simulink model "sim_project2"  (R2022a)
settings: Solver=VariableStepAuto  StartTime=0.0  StopTime=10.0  RelTol=1e-3
values from neighbouring files (symbols this model uses):
  A = A-B*Kctrl    [project.m]
  Ad = [0 0 0 0 0 0; 1 0 0 0 0 0; 2 1 0 0 0 0; 3 1 6 0 0 0; 1 2 1 3 0 0; 1 1 1 4 1 0]    [project.m]
  B = [0 -9.9453]'    [project.m]
  C = [708.27 0; 0 0]    [project.m]
  c = 10/(2*min(real(lam_g)))    [project.m]
  F = -F'    [project.m]
  G = diag([1 1 1 1 1 1])    [project.m]
  K = R^-1*B'*Pc    [project.m]
  Lun = Lun'    [project.m]
  n = length(B)    [project.m]
  noise = randn    [project.m]
  X0 = [10 2]'    [project.m]
settings Model: Creator=matildezampolini  LastModifiedBy=matildezampolini

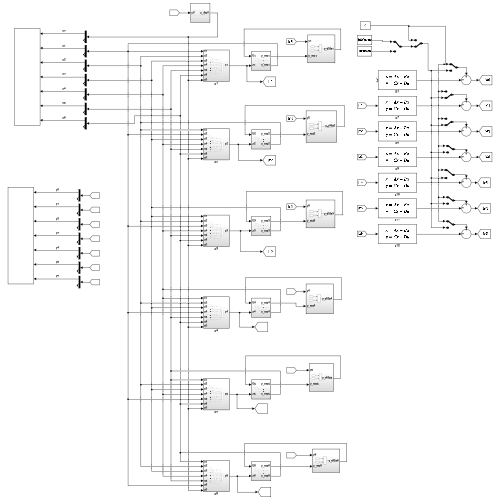
[thumbnail: Simulink's stored preview of the top-level diagram]
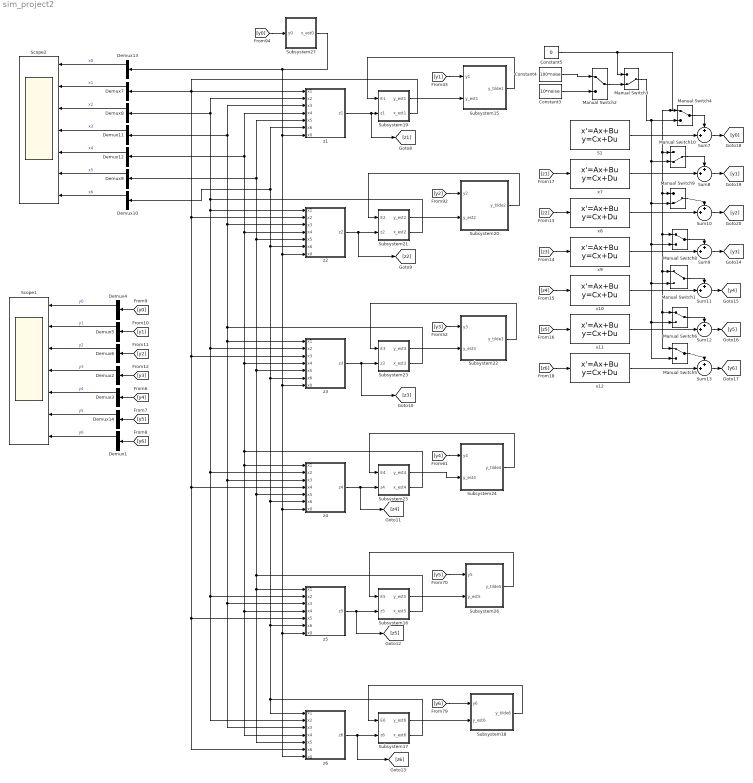
== system sim_project2 ==
  Constant3 : Constant  Value=10*noise
  Constant4 : Constant  Value=100*noise
  Constant5 : Constant  Value=0
  Demux{1..14} (14 alike) : Demux  Outputs=2
  Manual Switch{1..2,4..6,8} (6 alike) : ManualSwitch
  Manual Switch10 : ManualSwitch  CurrentSetting=0
  Manual Switch3 : ManualSwitch  CurrentSetting=0
  Manual Switch9 : ManualSwitch  CurrentSetting=0
  S1 : StateSpace  A=A  B=zeros(n,1)  C=C  D=zeros(n,1)  InitialCondition=X0
  Scope1 : Scope  NumInputPorts=7
  Scope2 : Scope  NumInputPorts=7
  Subsystem15 : Subsystem
  Subsystem16 : Subsystem
  Subsystem17 : Subsystem
  Subsystem18 : Subsystem
  Subsystem19 : Subsystem
  Subsystem20 : Subsystem
  Subsystem21 : Subsystem
  Subsystem22 : Subsystem
  Subsystem23 : Subsystem
  Subsystem24 : Subsystem
  Subsystem25 : Subsystem
  Subsystem26 : Subsystem
  Subsystem27 : Subsystem
  Sum{7..13} (7 alike) : Sum  Inputs=++|
  x{7..12} (6 alike) : StateSpace  A=A  B=c*B*K  C=C  D=zeros(n)  InitialCondition=0
  z1 : Subsystem
  z2 : Subsystem
  z3 : Subsystem
  z4 : Subsystem
  z5 : Subsystem
  z6 : Subsystem
  wires:
  [y4] -> Subsystem24/1(y4)
  Demux14/1 -> Scope1/6  "y5"
  Subsystem19/2(x_est1) -> Demux7/1, z2/2(x2), z5/5(x5), z6/6(x6), z4/4(x4), z3/3(x3), z1/1(x1)
  [y2] -> Demux6/1
  [y5] -> Subsystem26/1(y5)
  z5/1(z5) -> [z5], Subsystem16/2(z5)
  z1/1(z1) -> [z1], Subsystem19/2(z1)
  Subsystem25/1(y_est4) -> Subsystem24/2(y_est4)
  Demux4/1 -> Scope1/1  "y0"
  z6/1(z6) -> [z6], Subsystem17/2(z6)
  Demux5/1 -> Scope1/2  "y1"
  Demux3/1 -> Scope1/5  "y4"
  Subsystem25/2(x_est4) -> z3/4(x4), z2/4(x4), Demux12/1, z1/4(x4), z4/1(x1), z6/4(x4), z5/4(x4)
  Subsystem23/1(y_est3) -> Subsystem22/2(y_est3)
  Demux1/1 -> Scope1/7  "y6"
  Demux12/1 -> Scope2/5  "x4"
  Subsystem21/2(x_est2) -> z2/1(x1), z4/2(x2), z5/2(x2), z6/2(x2), z3/2(x2), z1/2(x2), Demux8/1
  Subsystem23/2(x_est3) -> z3/1(x1), z4/3(x3), z5/3(x3), z6/3(x3), z2/3(x3), Demux11/1, z1/3(x3)
  Demux9/1 -> Scope2/6  "x5"
  Demux6/1 -> Scope1/3  "y2"
  z4/1(z4) -> [z4], Subsystem25/2(z4)
  [y4] -> Demux3/1
  [y3] -> Demux2/1
  Demux2/1 -> Scope1/4  "y3"
  Subsystem16/1(y_est5) -> Subsystem26/2(y_est5)
  [y0] -> Demux4/1
  Subsystem17/2(x_est6) -> z5/6(x6), z3/6(x6), z2/6(x6), Demux10/1, z1/6(x6), z4/6(x6), z6/1(x1)
  [y6] -> Demux1/1
  [y1] -> Demux5/1
  [y5] -> Demux14/1
  Subsystem27/1(x_est0) -> z1/7(x0), z4/7(x0), z5/7(x0), z6/7(x0), z3/7(x0), z2/7(x0), Demux13/1
  [y1] -> Subsystem15/1(y1)
  Demux10/1 -> Scope2/7  "x6"
  Demux7/1 -> Scope2/2  "x1"
  Demux13/1 -> Scope2/1  "x0"
  [y3] -> Subsystem22/1(y3)
  Demux11/1 -> Scope2/4  "x3"
  [y2] -> Subsystem20/1(y2)
  Subsystem17/1(y_est6) -> Subsystem18/2(y_est6)
  Subsystem16/2(x_est5) -> z4/5(x5), z3/5(x5), z2/5(x5), z1/5(x5), Demux9/1, z5/1(x1), z6/5(x5)
  [y6] -> Subsystem18/1(y6)
  z3/1(z3) -> [z3], Subsystem23/2(z3)
  [y0] -> Subsystem27/1(y0)
  Subsystem21/1(y_est2) -> Subsystem20/2(y_est2)
  z2/1(z2) -> [z2], Subsystem21/2(z2)
  Demux8/1 -> Scope2/3  "x2"
  Subsystem19/1(y_est1) -> Subsystem15/2(y_est1)
  Subsystem15/1(y_tilde1) -> Subsystem19/1(E1)
  Subsystem20/1(y_tilde2) -> Subsystem21/1(E2)
  Subsystem22/1(y_tilde3) -> Subsystem23/1(E3)
  Subsystem24/1(y_tilde4) -> Subsystem25/1(E4)
  Subsystem26/1(y_tilde5) -> Subsystem16/1(E5)
  Subsystem18/1(y_tilde6) -> Subsystem17/1(E6)
  Manual Switch8/1 -> Sum9/1
  Sum8/1 -> [y1]
  [z4] -> x10/1
  Sum9/1 -> [y3]
  Sum10/1 -> [y2]
  [z5] -> x11/1
  Manual Switch4/1 -> Sum7/1
  [z2] -> x8/1
  Manual Switch10/1 -> Sum8/1
  Sum12/1 -> [y5]
  Manual Switch2/1 -> Manual Switch3/2
  [z3] -> x9/1
  Constant4/1 -> Manual Switch2/1
  Manual Switch3/1 -> Manual Switch4/2, Manual Switch8/2, Manual Switch1/2, Manual Switch6/2, Manual Switch5/2, Manual Switch9/2, Manual Switch10/2
  Manual Switch9/1 -> Sum10/1
  Manual Switch6/1 -> Sum12/1
  S1/1 -> Sum7/2
  x10/1 -> Sum11/2
  x12/1 -> Sum13/2
  [z6] -> x12/1
  x11/1 -> Sum12/2
  Manual Switch5/1 -> Sum13/1
  Manual Switch1/1 -> Sum11/1
  x7/1 -> Sum8/2
  Constant3/1 -> Manual Switch2/2
  x9/1 -> Sum9/2
  [z1] -> x7/1
  Constant5/1 -> Manual Switch1/1, Manual Switch5/1, Manual Switch6/1, Manual Switch8/1, Manual Switch9/1, Manual Switch10/1, Manual Switch4/1, Manual Switch3/1
  x8/1 -> Sum10/2
  Sum11/1 -> [y4]
  Sum7/1 -> [y0]
  Sum13/1 -> [y6]

== system sim_project2/Subsystem15 ==
  y1 : Inport
  y_est1 : Inport  Port=2
  Add2 : Sum  Inputs=+-
  y_tilde1 : Outport
  wires:
  Add2/1 -> y_tilde1/1
  y_est1/1 -> Add2/2
  y1/1 -> Add2/1

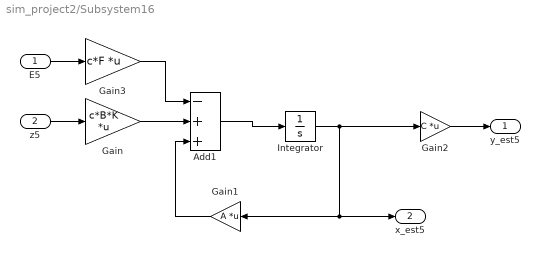
== system sim_project2/Subsystem16 ==
  E5 : Inport
  z5 : Inport  Port=2
  Add1 : Sum  Inputs=-++
  Gain : Gain  Gain=c*B*K  Multiplication=Matrix(K*u)
  Gain1 : Gain  Gain=A  Multiplication=Matrix(K*u)
  Gain2 : Gain  Gain=C  Multiplication=Matrix(K*u)
  Gain3 : Gain  Gain=c*F  Multiplication=Matrix(K*u)
  Integrator : Integrator
  y_est5 : Outport
  x_est5 : Outport  Port=2
  wires:
  Gain1/1 -> Add1/3
  E5/1 -> Gain3/1
  Add1/1 -> Integrator/1
  Gain3/1 -> Add1/1
  Gain2/1 -> y_est5/1
  Integrator/1 -> Gain2/1, x_est5/1, Gain1/1
  Gain/1 -> Add1/2
  z5/1 -> Gain/1

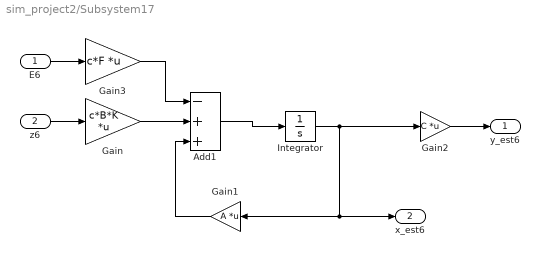
== system sim_project2/Subsystem17 ==
  E6 : Inport
  z6 : Inport  Port=2
  Add1 : Sum  Inputs=-++
  Gain : Gain  Gain=c*B*K  Multiplication=Matrix(K*u)
  Gain1 : Gain  Gain=A  Multiplication=Matrix(K*u)
  Gain2 : Gain  Gain=C  Multiplication=Matrix(K*u)
  Gain3 : Gain  Gain=c*F  Multiplication=Matrix(K*u)
  Integrator : Integrator
  y_est6 : Outport
  x_est6 : Outport  Port=2
  wires:
  Gain1/1 -> Add1/3
  E6/1 -> Gain3/1
  Add1/1 -> Integrator/1
  Gain3/1 -> Add1/1
  Gain2/1 -> y_est6/1
  Integrator/1 -> Gain2/1, x_est6/1, Gain1/1
  Gain/1 -> Add1/2
  z6/1 -> Gain/1

== system sim_project2/Subsystem18 ==
  y6 : Inport
  y_est6 : Inport  Port=2
  Add7 : Sum  Inputs=+-
  y_tilde6 : Outport
  wires:
  y_est6/1 -> Add7/2
  Add7/1 -> y_tilde6/1
  y6/1 -> Add7/1

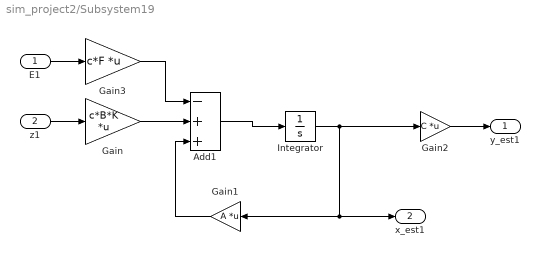
== system sim_project2/Subsystem19 ==
  E1 : Inport
  z1 : Inport  Port=2
  Add1 : Sum  Inputs=-++
  Gain : Gain  Gain=c*B*K  Multiplication=Matrix(K*u)
  Gain1 : Gain  Gain=A  Multiplication=Matrix(K*u)
  Gain2 : Gain  Gain=C  Multiplication=Matrix(K*u)
  Gain3 : Gain  Gain=c*F  Multiplication=Matrix(K*u)
  Integrator : Integrator
  y_est1 : Outport
  x_est1 : Outport  Port=2
  wires:
  E1/1 -> Gain3/1
  Add1/1 -> Integrator/1
  Gain3/1 -> Add1/1
  Gain2/1 -> y_est1/1
  Integrator/1 -> Gain2/1, x_est1/1, Gain1/1
  Gain/1 -> Add1/2
  z1/1 -> Gain/1
  Gain1/1 -> Add1/3

== system sim_project2/Subsystem20 ==
  y2 : Inport
  y_est2 : Inport  Port=2
  Add3 : Sum  Inputs=+-
  y_tilde2 : Outport
  wires:
  y_est2/1 -> Add3/2
  Add3/1 -> y_tilde2/1
  y2/1 -> Add3/1

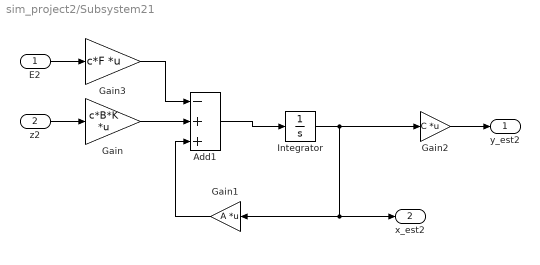
== system sim_project2/Subsystem21 ==
  E2 : Inport
  z2 : Inport  Port=2
  Add1 : Sum  Inputs=-++
  Gain : Gain  Gain=c*B*K  Multiplication=Matrix(K*u)
  Gain1 : Gain  Gain=A  Multiplication=Matrix(K*u)
  Gain2 : Gain  Gain=C  Multiplication=Matrix(K*u)
  Gain3 : Gain  Gain=c*F  Multiplication=Matrix(K*u)
  Integrator : Integrator
  y_est2 : Outport
  x_est2 : Outport  Port=2
  wires:
  E2/1 -> Gain3/1
  Add1/1 -> Integrator/1
  Gain3/1 -> Add1/1
  Gain2/1 -> y_est2/1
  Integrator/1 -> Gain2/1, x_est2/1, Gain1/1
  Gain/1 -> Add1/2
  z2/1 -> Gain/1
  Gain1/1 -> Add1/3

== system sim_project2/Subsystem22 ==
  y3 : Inport
  y_est3 : Inport  Port=2
  Add4 : Sum  Inputs=+-
  y_tilde3 : Outport
  wires:
  y_est3/1 -> Add4/2
  y3/1 -> Add4/1
  Add4/1 -> y_tilde3/1

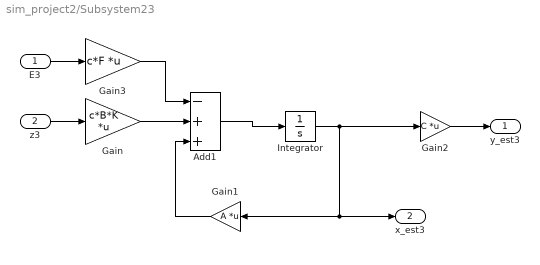
== system sim_project2/Subsystem23 ==
  E3 : Inport
  z3 : Inport  Port=2
  Add1 : Sum  Inputs=-++
  Gain : Gain  Gain=c*B*K  Multiplication=Matrix(K*u)
  Gain1 : Gain  Gain=A  Multiplication=Matrix(K*u)
  Gain2 : Gain  Gain=C  Multiplication=Matrix(K*u)
  Gain3 : Gain  Gain=c*F  Multiplication=Matrix(K*u)
  Integrator : Integrator
  y_est3 : Outport
  x_est3 : Outport  Port=2
  wires:
  E3/1 -> Gain3/1
  Add1/1 -> Integrator/1
  Gain3/1 -> Add1/1
  Gain2/1 -> y_est3/1
  Integrator/1 -> Gain2/1, x_est3/1, Gain1/1
  Gain/1 -> Add1/2
  z3/1 -> Gain/1
  Gain1/1 -> Add1/3

== system sim_project2/Subsystem24 ==
  y4 : Inport
  y_est4 : Inport  Port=2
  Add5 : Sum  Inputs=+-
  y_tilde4 : Outport
  wires:
  y_est4/1 -> Add5/2
  Add5/1 -> y_tilde4/1
  y4/1 -> Add5/1

== system sim_project2/Subsystem25 ==
  E4 : Inport
  z4 : Inport  Port=2
  Add1 : Sum  Inputs=-++
  Gain : Gain  Gain=c*B*K  Multiplication=Matrix(K*u)
  Gain1 : Gain  Gain=A  Multiplication=Matrix(K*u)
  Gain2 : Gain  Gain=C  Multiplication=Matrix(K*u)
  Gain3 : Gain  Gain=c*F  Multiplication=Matrix(K*u)
  Integrator : Integrator
  y_est4 : Outport
  x_est4 : Outport  Port=2
  wires:
  Gain1/1 -> Add1/3
  E4/1 -> Gain3/1
  Add1/1 -> Integrator/1
  Gain3/1 -> Add1/1
  Gain2/1 -> y_est4/1
  Integrator/1 -> Gain2/1, x_est4/1, Gain1/1
  Gain/1 -> Add1/2
  z4/1 -> Gain/1

== system sim_project2/Subsystem26 ==
  y5 : Inport
  y_est5 : Inport  Port=2
  Add6 : Sum  Inputs=+-
  y_tilde5 : Outport
  wires:
  Add6/1 -> y_tilde5/1
  y_est5/1 -> Add6/2
  y5/1 -> Add6/1

== system sim_project2/Subsystem27 ==
  y0 : Inport
  Add1 : Sum  Inputs=-+
  Add2 : Sum  Inputs=-+
  Gain1 : Gain  Gain=A  Multiplication=Matrix(K*u)
  Gain2 : Gain  Gain=C  Multiplication=Matrix(K*u)
  Gain4 : Gain  Gain=Lun  Multiplication=Matrix(K*u)
  Integrator : Integrator  InitialCondition=X0
  x_est0 : Outport
  wires:
  Add1/1 -> Integrator/1
  Gain2/1 -> Add2/2
  Integrator/1 -> Gain2/1, x_est0/1, Gain1/1
  y0/1 -> Add2/1
  Gain4/1 -> Add1/1
  Add2/1 -> Gain4/1
  Gain1/1 -> Add1/2

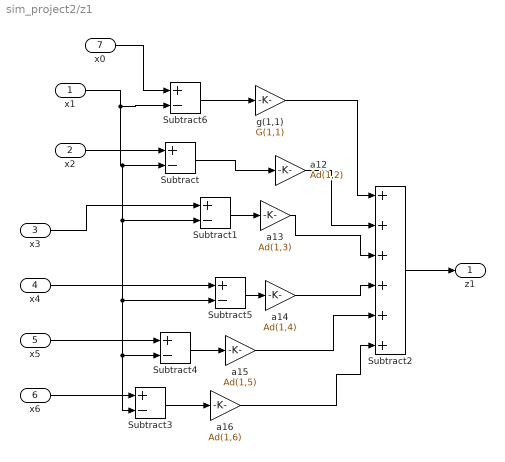
== system sim_project2/z1 ==
  x1 : Inport
  x2 : Inport  Port=2
  x3 : Inport  Port=3
  x4 : Inport  Port=4
  x5 : Inport  Port=5
  x6 : Inport  Port=6
  x0 : Inport  Port=7
  Subtract{,1,3..6} (6 alike) : Sum  Inputs=+-
  Subtract2 : Sum  Inputs=++++++
  a12 : Gain  Gain=Ad(1,2)
  a13 : Gain  Gain=Ad(1,3)
  a14 : Gain  Gain=Ad(1,4)
  a15 : Gain  Gain=Ad(1,5)
  a16 : Gain  Gain=Ad(1,6)
  g(1,1) : Gain  Gain=G(1,1)
  z1 : Outport
  wires:
  x2/1 -> Subtract/1
  x1/1 -> Subtract6/2, Subtract3/2, Subtract4/2, Subtract5/2, Subtract1/2, Subtract/2
  x3/1 -> Subtract1/1
  x4/1 -> Subtract5/1
  x5/1 -> Subtract4/1
  x6/1 -> Subtract3/1
  Subtract/1 -> a12/1
  Subtract1/1 -> a13/1
  Subtract5/1 -> a14/1
  Subtract4/1 -> a15/1
  Subtract3/1 -> a16/1
  a12/1 -> Subtract2/2
  a13/1 -> Subtract2/3
  a14/1 -> Subtract2/4
  a15/1 -> Subtract2/5
  a16/1 -> Subtract2/6
  Subtract2/1 -> z1/1
  x0/1 -> Subtract6/1
  Subtract6/1 -> g(1,1)/1
  g(1,1)/1 -> Subtract2/1

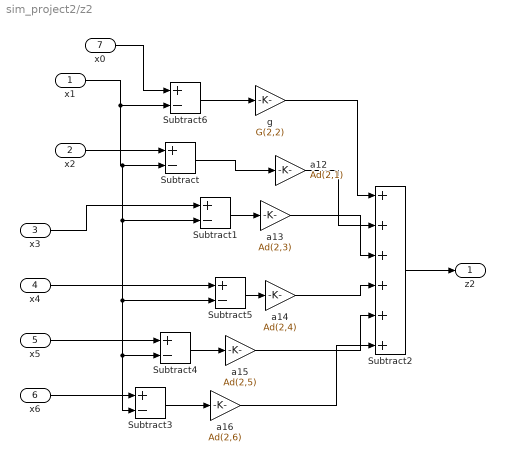
== system sim_project2/z2 ==
  x1 : Inport
  x2 : Inport  Port=2
  x3 : Inport  Port=3
  x4 : Inport  Port=4
  x5 : Inport  Port=5
  x6 : Inport  Port=6
  x0 : Inport  Port=7
  Subtract{,1,3..6} (6 alike) : Sum  Inputs=+-
  Subtract2 : Sum  Inputs=++++++
  a12 : Gain  Gain=Ad(2,1)
  a13 : Gain  Gain=Ad(2,3)
  a14 : Gain  Gain=Ad(2,4)
  a15 : Gain  Gain=Ad(2,5)
  a16 : Gain  Gain=Ad(2,6)
  g : Gain  Gain=G(2,2)
  z2 : Outport
  wires:
  x2/1 -> Subtract/1
  x1/1 -> Subtract3/2, Subtract4/2, Subtract5/2, Subtract1/2, Subtract/2, Subtract6/2
  x3/1 -> Subtract1/1
  x4/1 -> Subtract5/1
  x5/1 -> Subtract4/1
  x6/1 -> Subtract3/1
  Subtract/1 -> a12/1
  Subtract1/1 -> a13/1
  Subtract5/1 -> a14/1
  Subtract4/1 -> a15/1
  Subtract3/1 -> a16/1
  a12/1 -> Subtract2/2
  a13/1 -> Subtract2/3
  a14/1 -> Subtract2/4
  a15/1 -> Subtract2/5
  a16/1 -> Subtract2/6
  Subtract2/1 -> z2/1
  x0/1 -> Subtract6/1
  Subtract6/1 -> g/1
  g/1 -> Subtract2/1

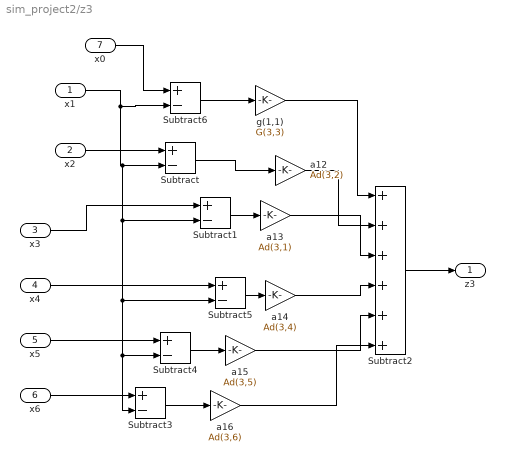
== system sim_project2/z3 ==
  x1 : Inport
  x2 : Inport  Port=2
  x3 : Inport  Port=3
  x4 : Inport  Port=4
  x5 : Inport  Port=5
  x6 : Inport  Port=6
  x0 : Inport  Port=7
  Subtract{,1,3..6} (6 alike) : Sum  Inputs=+-
  Subtract2 : Sum  Inputs=++++++
  a12 : Gain  Gain=Ad(3,2)
  a13 : Gain  Gain=Ad(3,1)
  a14 : Gain  Gain=Ad(3,4)
  a15 : Gain  Gain=Ad(3,5)
  a16 : Gain  Gain=Ad(3,6)
  g(1,1) : Gain  Gain=G(3,3)
  z3 : Outport
  wires:
  x2/1 -> Subtract/1
  x1/1 -> Subtract6/2, Subtract3/2, Subtract4/2, Subtract5/2, Subtract1/2, Subtract/2
  x3/1 -> Subtract1/1
  x4/1 -> Subtract5/1
  x5/1 -> Subtract4/1
  x6/1 -> Subtract3/1
  Subtract/1 -> a12/1
  Subtract1/1 -> a13/1
  Subtract5/1 -> a14/1
  Subtract4/1 -> a15/1
  Subtract3/1 -> a16/1
  a12/1 -> Subtract2/2
  a13/1 -> Subtract2/3
  a14/1 -> Subtract2/4
  a15/1 -> Subtract2/5
  a16/1 -> Subtract2/6
  Subtract2/1 -> z3/1
  x0/1 -> Subtract6/1
  Subtract6/1 -> g(1,1)/1
  g(1,1)/1 -> Subtract2/1

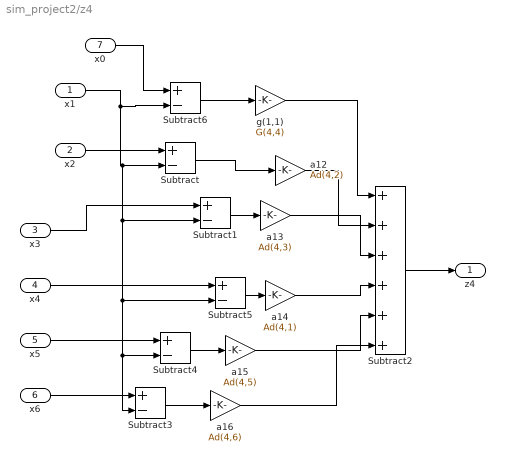
== system sim_project2/z4 ==
  x1 : Inport
  x2 : Inport  Port=2
  x3 : Inport  Port=3
  x4 : Inport  Port=4
  x5 : Inport  Port=5
  x6 : Inport  Port=6
  x0 : Inport  Port=7
  Subtract{,1,3..6} (6 alike) : Sum  Inputs=+-
  Subtract2 : Sum  Inputs=++++++
  a12 : Gain  Gain=Ad(4,2)
  a13 : Gain  Gain=Ad(4,3)
  a14 : Gain  Gain=Ad(4,1)
  a15 : Gain  Gain=Ad(4,5)
  a16 : Gain  Gain=Ad(4,6)
  g(1,1) : Gain  Gain=G(4,4)
  z4 : Outport
  wires:
  x2/1 -> Subtract/1
  x1/1 -> Subtract6/2, Subtract3/2, Subtract4/2, Subtract5/2, Subtract1/2, Subtract/2
  x3/1 -> Subtract1/1
  x4/1 -> Subtract5/1
  x5/1 -> Subtract4/1
  x6/1 -> Subtract3/1
  Subtract/1 -> a12/1
  Subtract1/1 -> a13/1
  Subtract5/1 -> a14/1
  Subtract4/1 -> a15/1
  Subtract3/1 -> a16/1
  a12/1 -> Subtract2/2
  a13/1 -> Subtract2/3
  a14/1 -> Subtract2/4
  a15/1 -> Subtract2/5
  a16/1 -> Subtract2/6
  Subtract2/1 -> z4/1
  x0/1 -> Subtract6/1
  Subtract6/1 -> g(1,1)/1
  g(1,1)/1 -> Subtract2/1

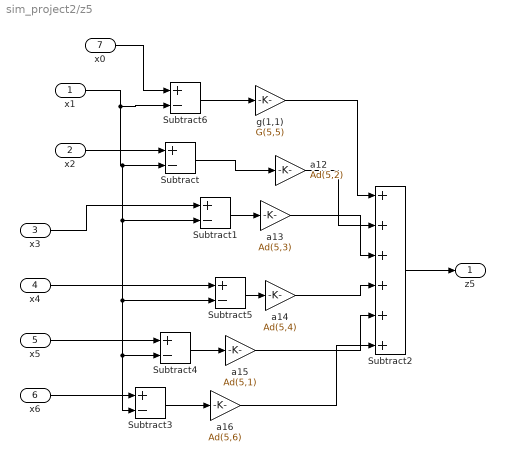
== system sim_project2/z5 ==
  x1 : Inport
  x2 : Inport  Port=2
  x3 : Inport  Port=3
  x4 : Inport  Port=4
  x5 : Inport  Port=5
  x6 : Inport  Port=6
  x0 : Inport  Port=7
  Subtract{,1,3..6} (6 alike) : Sum  Inputs=+-
  Subtract2 : Sum  Inputs=++++++
  a12 : Gain  Gain=Ad(5,2)
  a13 : Gain  Gain=Ad(5,3)
  a14 : Gain  Gain=Ad(5,4)
  a15 : Gain  Gain=Ad(5,1)
  a16 : Gain  Gain=Ad(5,6)
  g(1,1) : Gain  Gain=G(5,5)
  z5 : Outport
  wires:
  x2/1 -> Subtract/1
  x1/1 -> Subtract6/2, Subtract3/2, Subtract4/2, Subtract5/2, Subtract1/2, Subtract/2
  x3/1 -> Subtract1/1
  x4/1 -> Subtract5/1
  x5/1 -> Subtract4/1
  x6/1 -> Subtract3/1
  Subtract/1 -> a12/1
  Subtract1/1 -> a13/1
  Subtract5/1 -> a14/1
  Subtract4/1 -> a15/1
  Subtract3/1 -> a16/1
  a12/1 -> Subtract2/2
  a13/1 -> Subtract2/3
  a14/1 -> Subtract2/4
  a15/1 -> Subtract2/5
  a16/1 -> Subtract2/6
  Subtract2/1 -> z5/1
  x0/1 -> Subtract6/1
  Subtract6/1 -> g(1,1)/1
  g(1,1)/1 -> Subtract2/1

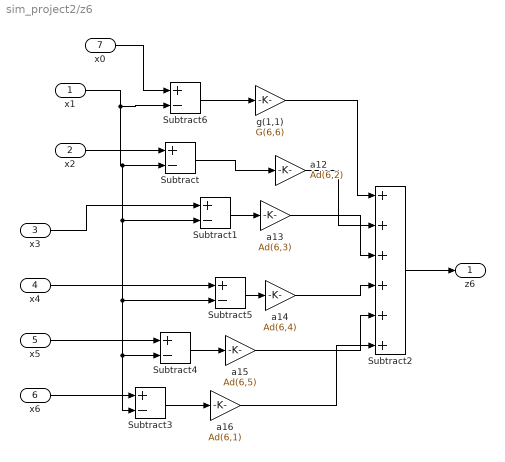
== system sim_project2/z6 ==
  x1 : Inport
  x2 : Inport  Port=2
  x3 : Inport  Port=3
  x4 : Inport  Port=4
  x5 : Inport  Port=5
  x6 : Inport  Port=6
  x0 : Inport  Port=7
  Subtract{,1,3..6} (6 alike) : Sum  Inputs=+-
  Subtract2 : Sum  Inputs=++++++
  a12 : Gain  Gain=Ad(6,2)
  a13 : Gain  Gain=Ad(6,3)
  a14 : Gain  Gain=Ad(6,4)
  a15 : Gain  Gain=Ad(6,5)
  a16 : Gain  Gain=Ad(6,1)
  g(1,1) : Gain  Gain=G(6,6)
  z6 : Outport
  wires:
  x2/1 -> Subtract/1
  x1/1 -> Subtract6/2, Subtract3/2, Subtract4/2, Subtract5/2, Subtract1/2, Subtract/2
  x3/1 -> Subtract1/1
  x4/1 -> Subtract5/1
  x5/1 -> Subtract4/1
  x6/1 -> Subtract3/1
  Subtract/1 -> a12/1
  Subtract1/1 -> a13/1
  Subtract5/1 -> a14/1
  Subtract4/1 -> a15/1
  Subtract3/1 -> a16/1
  a12/1 -> Subtract2/2
  a13/1 -> Subtract2/3
  a14/1 -> Subtract2/4
  a15/1 -> Subtract2/5
  a16/1 -> Subtract2/6
  Subtract2/1 -> z6/1
  x0/1 -> Subtract6/1
  Subtract6/1 -> g(1,1)/1
  g(1,1)/1 -> Subtract2/1
